simulink model "mathematical_modeling"  (R2017b)
settings: Solver=VariableStepAuto  StartTime=0.0  StopTime=10.0  RelTol=1e-3
settings Model: Creator=Damla  LastModifiedBy=dagac

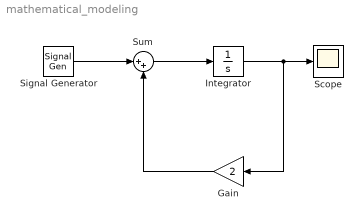
== system mathematical_modeling ==
  Gain : Gain  Gain=2
  Integrator : Integrator
  Scope : Scope
  Signal Generator : SignalGenerator  WaveForm=square
  Sum : Sum  Inputs=|++
  wires:
  Signal Generator/1 -> Sum/1
  Gain/1 -> Sum/2
  Sum/1 -> Integrator/1
  Integrator/1 -> Scope/1, Gain/1
